simulink model "spread_spectrum"  (R2023b)
settings: Solver=VariableStepAuto  StartTime=0.0  StopTime=10.0  RelTol=1e-3
libraries: commdigbbndpm3 x3, commrandsrc3 x1
settings Model: Creator=Biancaa. R  LastModifiedBy=Biancaa. R

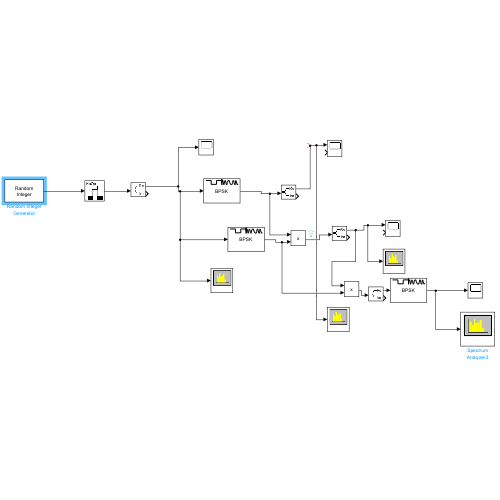
[thumbnail: Simulink's stored preview of the top-level diagram]
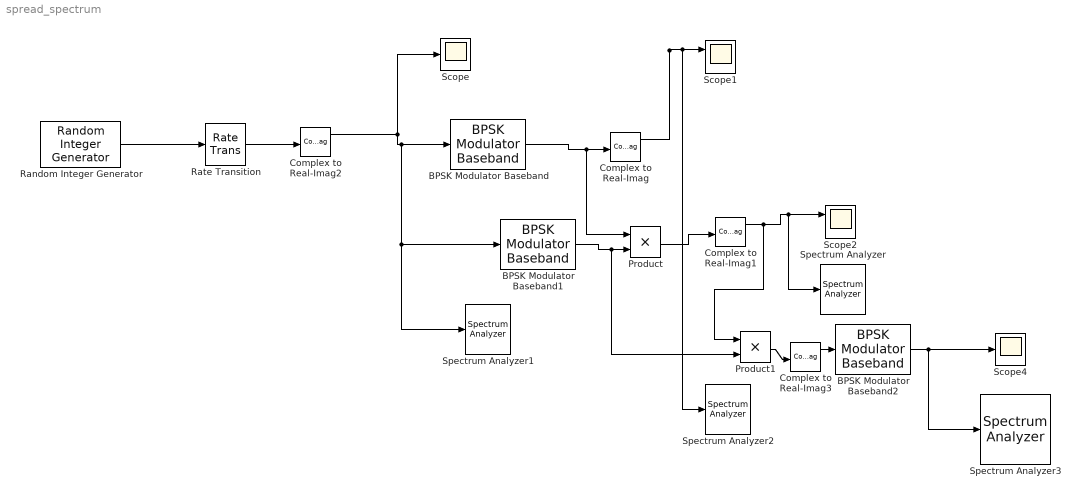
== system spread_spectrum ==
  BPSK Modulator Baseband : commdigbbndpm3/BPSK Modulator Baseband  Ph=0  outDtype=double  outWordLen=16  outUDDataType=sfix(16)  outFracLenMode=Best precision  outFracLen=15  outDataTypeStr=double  outLastDataTypeStr=double
  BPSK Modulator Baseband1 : commdigbbndpm3/BPSK Modulator Baseband  Ph=0  outDtype=double  outWordLen=16  outUDDataType=sfix(16)  outFracLenMode=Best precision  outFracLen=15  outDataTypeStr=double  outLastDataTypeStr=double
  BPSK Modulator Baseband2 : commdigbbndpm3/BPSK Modulator Baseband  Ph=0  outDtype=double  outWordLen=16  outUDDataType=sfix(16)  outFracLenMode=Best precision  outFracLen=15  outDataTypeStr=double  outLastDataTypeStr=double
  Complex to Real-Imag{,1..3} (4 alike) : ComplexToRealImag
  Product : Product
  Product1 : Product
  Random Integer Generator : commrandsrc3/Random Integer Generator  SetSize=1023  SeedSource=Auto  Seed=0  SampleTime=1  SamplesPerFrame=1  OutputDataType=uint32  SimulateUsing=Interpreted execution
  Rate Transition : RateTransition
  Scope : Scope
  Scope1 : Scope  NumInputPorts=2
  Scope2 : Scope  NumInputPorts=2
  Scope4 : Scope
  Spectrum Analyzer{,1..3} (4 alike) : SpectrumAnalyzer  WindowPosition=[368.000000,182.000000,800.000000,500.000000,]  ScopeFrameLocation=window
  wires:
  Random Integer Generator/1 -> Rate Transition/1
  BPSK Modulator Baseband/1 -> Product/1, Complex to Real-Imag/1
  Complex to Real-Imag/1 -> Scope1/1, Spectrum Analyzer2/1
  BPSK Modulator Baseband1/1 -> Product1/2, Product/2
  Product/1 -> Complex to Real-Imag1/1
  Complex to Real-Imag1/1 -> Product1/1, Spectrum Analyzer/1, Scope2/1
  BPSK Modulator Baseband2/1 -> Spectrum Analyzer3/1, Scope4/1
  Rate Transition/1 -> Complex to Real-Imag2/1
  Complex to Real-Imag2/1 -> Spectrum Analyzer1/1, BPSK Modulator Baseband1/1, BPSK Modulator Baseband/1, Scope/1
  Complex to Real-Imag3/1 -> BPSK Modulator Baseband2/1
  Product1/1 -> Complex to Real-Imag3/1
